simulink model "clrrtsf"  (R2020a)
settings: Solver=FixedStepAuto  StartTime=0.0  StopTime=inf  FixedStep=0.2  RelTol=1e-3
model workspace (MAT data in the model file):
  IC_theta0 : Simulink.Signal (value not decoded)
  IC_x0 : Simulink.Signal (value not decoded)
  IC_x1 : Simulink.Signal (value not decoded)
  IC_y0 : Simulink.Signal (value not decoded)
  IC_y1 : Simulink.Signal (value not decoded)
  contsim_time : Simulink.Signal (value not decoded)
  indicator : Simulink.Signal (value not decoded)
  ip : Simulink.Signal (value not decoded)
  szxx1 : Simulink.Signal (value not decoded)
values from neighbouring files (symbols this model uses):
  indsimtime = 150    [clrrtsf_Initializ.m]
  L_0b = 0.48    [clrrtsf_Initializ.m]    (also in clrrtsolutionplot.m)
  L_0f = 3.8    [clrrtsf_Initializ.m]    (also in clrrtsolutionplot.m)
  L_1f = 7.21    [clrrtsf_Initializ.m]    (also in clrrtsolutionplot.m)
  LD = 10    [clrrtsf_Initializ.m]
  pinit = [80 160 pi 0]    [clrrtsf_Initializ.m]
  tn = zeros(N,14)    [clrrtsf_Initializ.m]    (also in clrrtsolutionplot.m = out.tree)
  veh_path = zeros(indsimtime,6)    [clrrtsf_Initializ.m]
  veh_path_col = zeros(indsimtime,6,N)    [clrrtsf_Initializ.m]
  xx = [-50:0.5:50]'    [clrrtsf_Initializ.m]
  yy = [-50:0.5:50]'    [clrrtsf_Initializ.m]
  Zf = griddata(x,y,znew,xnewt,ynewt)    [clrrtsf_Initializ.m]
  Zr = griddata(x,y,znewr,xnewt,ynewt)    [clrrtsf_Initializ.m]
symbols that are objects in the model workspace (value not decoded): IC_theta0, IC_x0, IC_x1, IC_y0, IC_y1
undefined symbols (not defined in the file or in its folder): DiscIntNeverNeededParam, IC_theta1
libraries: simulink x1
(part 2 of 2)

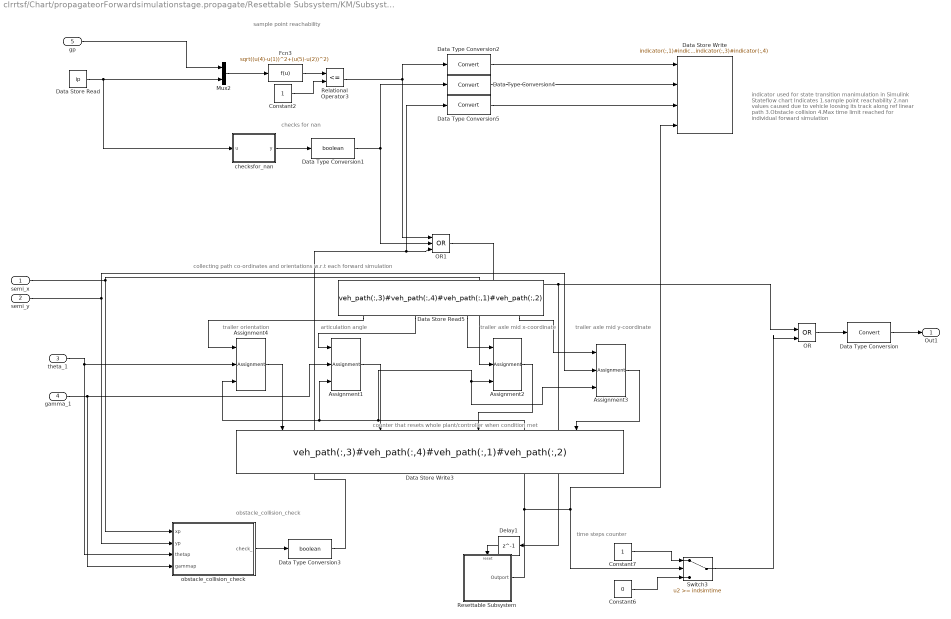
== system clrrtsf/Chart/propagateorForwardsimulationstage.propagate/Resettable Subsystem/KM/Subsystem ==
  note: indicator used for state transition
      | manimulation in Simulink Stateflow chart
      | Indicates
      | 1.sample point reachability
      | 2.nan values caused due to vehicle loosing its track
      | along ref linear path
      | 3.Obstacle collision
      | 4.Max time limit reached for individual forward simulation
  note: collecting path co-ordinates and orientations w.r.t each forward simulation
  note: time steps counter
  note: obstacle_collision_check
  note: counter that resets whole plant/controller when condition met
  note: checks for nan
  note: sample point reachability
  note: trailer axle mid x-coordinate
  note: trailer orientation
  note: articulation angle
  note: trailer axle mid y-coordinate
  semi_x : Inport
  semi_y : Inport  Port=2
  theta_1 : Inport  Port=3
  gamma_1 : Inport  Port=4  OutDataTypeStr=double  PortDimensions=1
  gp : Inport  Port=5
  Assignment{1..4} (4 alike) : Assignment  NumberOfDimensions=2  DiagnosticForDimensions=Warning  IndexOptions=Index vector (port),Index vector (dialog)  Indices=1,1  OutputSizes=1,1
  Constant2 : Constant
  Constant6 : Constant  Value=0
  Constant7 : Constant
  Data Store Read : DataStoreRead  DataStoreName=ip
  Data Store Read5 : DataStoreRead  DataStoreName=veh_path  DataStoreElements=veh_path(:,3)#veh_path(:,4)#veh_path(:,1)#veh_path(:,2)
  Data Store Write : DataStoreWrite  DataStoreName=indicator  DataStoreElements=indicator(:,1)#indicator(:,2)#indicator(:,3)#indicator(:,4)
  Data Store Write3 : DataStoreWrite  DataStoreName=veh_path  DataStoreElements=veh_path(:,3)#veh_path(:,4)#veh_path(:,1)#veh_path(:,2)
  Data Type Conversion{,2,4..5} (4 alike) : DataTypeConversion
  Data Type Conversion1 : DataTypeConversion  OutDataTypeStr=boolean
  Data Type Conversion3 : DataTypeConversion  OutDataTypeStr=boolean
  Delay1 : Delay  DelayLength=1
  Fcn3 : Fcn  Expr=sqrt((u(4)-u(1))^2+(u(5)-u(2))^2)
  Mux2 : Mux  Inputs=2
  OR : Logic  Operator=OR  IconShape=distinctive  AllPortsSameDT=off  OutDataTypeStr=boolean
  OR1 : Logic  Operator=OR  Inputs=3  IconShape=distinctive  AllPortsSameDT=off  OutDataTypeStr=boolean
  Relational Operator3 : RelationalOperator  Operator=<=  OutDataTypeStr=boolean  RndMeth=Simplest
  Resettable Subsystem : Subsystem  TreatAsAtomicUnit=on
  Switch3 : Switch  Threshold=indsimtime
  checksfor_nan : MATLAB Function  TreatAsAtomicUnit=on
  obstacle_collision_check : MATLAB Function  TreatAsAtomicUnit=on
  Out1 : Outport
  wires:
  Delay1/1 -> Resettable Subsystem/Reset
  Assignment2/1 -> Data Store Write3/3
  Constant6/1 -> Switch3/3
  Constant7/1 -> Switch3/1
  OR/1 -> Data Type Conversion/1
  Switch3/1 -> OR/2
  OR1/1 -> OR/1, Delay1/1
  Data Type Conversion/1 -> Out1/1
  semi_x/1 -> obstacle_collision_check/1(xp), Assignment2/2
  Data Store Read5/1 -> Assignment4/1
  Assignment4/1 -> Data Store Write3/1
  theta_1/1 -> obstacle_collision_check/3(thetap), Assignment4/2
  Assignment3/1 -> Data Store Write3/4
  Data Store Read/1 -> checksfor_nan/1(u), Mux2/2
  Fcn3/1 -> Relational Operator3/1
  gp/1 -> Mux2/1
  Constant2/1 -> Relational Operator3/2
  Mux2/1 -> Fcn3/1
  Relational Operator3/1 -> OR1/1, Data Type Conversion2/1
  checksfor_nan/1(y) -> Data Type Conversion1/1
  Data Type Conversion1/1 -> OR1/2, Data Type Conversion4/1
  obstacle_collision_check/1(check_) -> Data Type Conversion3/1
  Data Type Conversion3/1 -> Data Type Conversion5/1, OR1/3
  semi_y/1 -> obstacle_collision_check/2(yp), Assignment3/2
  gamma_1/1 -> obstacle_collision_check/4(gammap), Assignment1/2
  Resettable Subsystem/1(Outport) -> Data Store Write/4, Switch3/2, Assignment1/3, Assignment4/3, Assignment3/3, Assignment2/3
  Data Type Conversion2/1 -> Data Store Write/1
  Data Type Conversion4/1 -> Data Store Write/2
  Data Type Conversion5/1 -> Data Store Write/3
  Assignment1/1 -> Data Store Write3/2
  Data Store Read5/2 -> Assignment1/1
  Data Store Read5/3 -> Assignment2/1
  Data Store Read5/4 -> Assignment3/1

== system clrrtsf/Chart/propagateorForwardsimulationstage.propagate/Resettable Subsystem/KM/Subsystem/Resettable Subsystem ==
  Reset : ResetPort  DisableCoverage=on
  Add1 : Sum
  Constant2 : Constant
  Counter Limited : simulink/Sources/Counter Limited  uplimit=indsimtime-1  tsamp=-1
  Outport : Outport
  wires:
  Counter Limited/1 -> Add1/1
  Constant2/1 -> Add1/2
  Add1/1 -> Outport/1

== matlab function clrrtsf/Chart/stage1.f/For Iterator Subsystem/Subsystem/MATLAB Function1 ==
  data: Nn3 input; localco_ord output size=[1 2]; s input double size=[1 2]; tn data_store_memory
    function localco_ord=coordtransform(Nn3,s)
    global tn
    tnc=tn;
        %theta=90;
        alfa=zeros(1,1);
        if Nn3==1
         %calculating sampled point wrt local coordinates of Nn
            tx = s(1,1);
            ty = s(1,2);
            localco_ord=[tx ty];
        else

            %origin shift and axis rotate
            % - calculate theta is the angle between global X axis and line made by points t(i-1) and t(i)=s()
            % alfa angle btwn global Y axis and line made by points t(i-1) and t(i)=s()
            %            u=(Nn2-tn((Nn3-1),2));
            u=tnc((Nn3),2)- tnc((tnc((Nn3),4)),2);
            v=tnc((Nn3),1)- tnc((tnc((Nn3),4)),1);
            %             v=(Nn1-tn((Nn3-1),1));
            su=sign(u);
            sv=sign(v);
            m=(u)/(v);
            if su >0 && sv>0
                theta=atan(m)*(180/pi);
                alfa = -1*(90 - theta);%cw %270+theta ccw
            elseif su >0 && sv<0
                theta=(atan(m)*(180/pi))+180;    
                alfa=(theta-90);    %ccw
            elseif su <0 && sv<0
                theta=(atan(m)*(180/pi))+180;
                alfa = theta-90; %ccw
            elseif su <0 && sv>0
                theta=(atan(m)*(180/pi))+360; 
                alfa=theta-90; %ccw  %-90-1*(360-theta)cw %
            end
            %calculating sampled point wrt local coordinates of Nn
            tx = (cosd(alfa)*(s(1,1)-tnc((Nn3),1))+sind(alfa)*(s(1,2)-tnc((Nn3),2)));
            ty = (cosd(alfa)*(s(1,2)-tnc((Nn3),2))-sind(alfa)*(s(1,1)-tnc((Nn3),1)));
            localco_ord=[tx ty];
        end
    end

== matlab function clrrtsf/Chart/propagateorForwardsimulationstage.propagate/Resettable Subsystem/Controller/purepursuit_contrroller/func to calculate points of intersections ==
  data: gp input; Nn_ input; tn input; R input; P output; pos input
function P = calc_ips(gp, Nn_, tn, R,pos)
%this func calculates points of intersection between ref line (formed
%with goal point, start point) and look ahead circle with center at semitrailer axel midpoint  
P=zeros(2,2);
%
p1=gp;
p2=[tn(Nn_,1) tn(Nn_,2)];
slope = (p1(1,2)-p2(1,2))/(p1(1,1)-p2(1,1));
if slope == -inf || slope ==inf
    intercpt=p1(1,1);
else
intercpt = p2(1,2)-slope*p2(1,1);
end
%updating center of circle with the current pose of semitrailer axle
%position
centerx=pos(1,1);
centery=pos(2,1);
radius=R;
coder.extrinsic('linecirc')
[xout,yout] = linecirc(slope,intercpt,centerx,centery,radius);
P=[xout ; yout];

== stateflow chart clrrtsf/Chart ==
  note: Implementation of the CL-RRT algorithm in STATEFLOW
  note: START
  state logic for inverting stype variable [group]
    (junction 268) -> (junction 269) [order 1] : [stype==0]
    (junction 268) -> (junction 270) [order 2]
    (junction 269) -> (junction 274) : {stype=1;}
    (junction 270) -> (junction 271) [order 1] : [stype==1]
    (junction 270) -> (junction 272) [order 2]
    (junction 271) -> (junction 273) : {stype=0;}
    (junction 273) -> (junction 272)
    (junction 274) -> (junction 273)
    (junction 272) -> (junction 300) [order 2]
  state stage1
    en:
    %Random sampling when stype is 0
    [sr, v_0]= sampling(i,stype);
    %choosing between nearest and cheapest node with
    % probability of 0.5 for each case
    j=j+1;
    rnum=randnum(j,1);
    if  rnum<=0.5
    %cheapest node finder: f_()
    Nn_= f_(sr,i);
    else
    %Nearest node finder: f()
    Nn_=f(sr,i);
    end
    %Nn_ is the node number of current start point,
    %is uded to index into tree to find respective co-ordinates
    %assigning random sample as current goal point
    gp_(1,1:2)=sr;
    gp_(1,3)=0;%theta;
    % pice wise linear refpath creation between start and
    %goal points
    state Nn = f_(sr,i) [function]
    state Nn = f(sr,i) [function]
  state treebuilder
    i=i+1;   %node increment, where i is the current node number
    j = 0;
    if i==1
    Initialize();
    %initializing vehicle, controller parameters
    %tree, sampling type variable (stype),
    %individual traversedpath, collection of traversed paths
    %insert rootnode into tree
    else
    %parent node number
    pnode=Nn_;
    %m is a function that enters data into the tree array tn
    m(i,pnode,stype,v_0,goalregion);
    %calculating cumulative cost of the traversed path
    cumilativecost(i);
    end
    state cumilativecost(i) [function]
    state Initialize [function]
    state m(i,pnode,stype,f_or_r,goalregion) [function]
  state stage2
    en:
    %goal sampling when stype is 1
    [sg, v_0]= sampling(i,stype);
    % pice wise linear refpath creation
    %assigning goal sample as a
    %next goal point
    gp_(1,1:2)=sg;
    gp_(1,3)=0;%theta;
    %Nn_ is the node number of current
    %start point, is used to index into
    %tree to find respective co-ordinates
    Nn_=i;
    % pice wise linear refpath creation
    % between start and goal points
  state output_to_workspace
    %outputting the tree tn
    %of size Nx14
    %and traversed paths
    %collection in data store
    %with name
    %"Veh_path_col"
    output1wpace();
    state output1wpace [function]
  state updateInitialConfigurationofcontrollerwithNn_
    en:
    %updating the current
    %vehicle position to
    %controller
    updateICofcont(Nn_)
    state updateICofcont(Nn_) [function]
  state goalregion_reachability
    goalregion = goalregionreachability(pgoal);
    %pgoal is the final desired goal pose
    state goalregion = goalregionreachability(pgoal) [function]
  state stopsimulation
  state costcalculation
    en:
    %calculating cost of
    %individual traversed
    % paths by semitrailer
    % driveaxle mid point
    costcal(i);
    state costcal(i) [function]
  state propagateorForwardsimulationstage
    en:
    du:
    propagate(v_0,gp_,Nn_)
    state propagate(v_0,gp,Nn_) [function]
  note: STOP
  note: v_0 & v_1are the logotudinal velocity of tractor and semitrailer set to 1m/s; stype is a variable used to select random sample, (sr) or goal sample, (sg) within the sampling();
      | trans1 is the variable that indicates end of individual forward simulation; Indicator size 1x4 contains boolean values representing true false for sample point reachability, nan
      | values that might result due kinematic infeasibility,obstacle collision and maxtimelimit reach set for each individual forward simulation. Any of these four factors can stop the
      | individual simulation and continue to next; numofnodes is maxlimit on number of nodes
  (default) -> treebuilder : {i=0; rootnode=[190 187 pi 0 0 0 0 0];}
  treebuilder -> (junction 268) [order 2] : [i<numofnodes]
  (junction 272) -> (junction 218) [order 1]
  (junction 218) -> stage1 [order 1] : [ stype == 0]
  (junction 218) -> stage2 [order 2] : [stype == 1]
  treebuilder -> output_to_workspace [order 1] : [i>=numofnodes]
  (junction 242) -> stage1 [order 2] : [(indicator(1,4)<2 && indicator(1,3)==1) || (indicator(1,4)<2 && indicator(1,2)==1) ]
  stage1 -> updateInitialConfigurationofcontrollerwithNn_
  stage2 -> updateInitialConfigurationofcontrollerwithNn_
  output_to_workspace -> stopsimulation
  costcalculation -> treebuilder
  (junction 223) -> treebuilder [order 2] : [i>=numofnodes]
  updateInitialConfigurationofcontrollerwithNn_ -> propagateorForwardsimulationstage
  (junction 223) -> costcalculation [order 1] : [i<numofnodes]
  goalregion_reachability -> (junction 223)
  (junction 242) -> (junction 223) [order 3] : {goalregion=false;}
  (junction 242) -> goalregion_reachability [order 1] : [stype==1 && indicator(1,1)==1]
  propagateorForwardsimulationstage -> (junction 242) : [trans1==1]
  data: sr function_input double size=[1 2]; Nn function_output double; i function_input double size=1; sr function_input double size=[1 2]; Nn function_output double; i function_input double size=1; i function_input double size=[1 1]; i function_input double size=1; pnode function_input double size=1; stype function_input double size=[1 1]; f_or_r function_input double size=[1 1]; goalregion function_input double size=1; in function_input; stype_ function_input; s function_output; v_0_ function_output; Nn_ function_input double size=1; pgoal function_input double size=[1 3]; goalregion function_output; sf_internal_action_state_placeholder_data local double size=1 =0; i function_input double size=[1 1]; v_0 function_input double size=1; gp function_input double size=[1 3]; Nn_ function_input double size=1; tn data_store_memory; sr local size=[1 2]; gp_ local double size=[1 3]; Nn_ local double size=[1 1] =0; i local double size=[1 1] =1; rootnode local; stype local =1; pnode local =0; v_0 data_store_memory; numofnodes data_store_memory =300; sg local; trans1 data_store_memory; pgoal data_store_memory =[0 40 pi/2]; theta local double size=1; indicator data_store_memory; goalregion local; randnum data_store_memory; rnum local; j local
  function [s,v_0_] = sampling(in,stype_):
    | function [s,v_0_] = sampling(in,stype_)
    | %single function called sampling()is used to achive both random sampling ,
    | %(exploring strategy) and goal sampling (biasing strategy). The variable
    | %stype is used to choose the type of the sampling. 0 for random sampling,1
    | %for goal sampling
    | global tn
    | global pgoal
    | global randnum
    | 
    | persistent j
    | if isempty(j)
    | %  costarray=zeros(n,2);
    |  j=0;
    | end
    | j=j+1;
    | tnc=tn;
    | stype=stype_;
    | %rng('shuffle');
    | %rng ( 'default' );
    | while true
    | s=zeros(1,2);
    | v_0_=zeros(1,1);
    | n1=zeros(1,1);
    | refp1=[pgoal(1,1) 145];
    | refp2=[pgoal(1,1) 145];
    |  if stype==0  %random sampling     
    |             %n=rand;
    |             n=randnum(j,1);
    |             if (n>=0)&&(n<=0.2)
    |                 n1=1;
    |             elseif (n>0.2)&&(n<=0.7)
    |                 n1=2;
    |             elseif (n>0.7)&&(n<=1)
    |                 n1=3;
    |             end
    |             switch n1
    |                 case 1
    |                     %forward
    |                     sigmaU=[5,5];
    |                     %s(1,1)=tn(in,1)+ sqrt(3)*sigmaU(1)*(-1+2.*rand); %-1+2.*
    |                     s(1,1)=refp2(1,1)+ sqrt(3)*sigmaU(1)*(-1+2.*rand);
    |                     %s(1,2)=tn(in,2)+ sqrt(3)*sigmaU(2)*(-1+2.*rand); %-1+2.*
    |                     s(1,2)=refp2(1,2)+ sqrt(3)*sigmaU(2)*(-1+2.*rand);
    |                     v_0_=-1;
    |                 case 2
    |                     sigmaU=[2.5,5];
    |                     %s(1,1)=tn(in,1)+ sqrt(3)*sigmaU(1)*(-1+2.*rand); %-1+2.*
    |                     s(1,1)=refp2(1,1)+ sqrt(3)*sigmaU(1)*(-1+2.*rand);
    |                     %s(1,2)=tn(in,2)+ sqrt(3)*sigmaU(2)*(-1+2.*rand); %-1+2.*
    |                     s(1,2)=refp2(1,2)+ sqrt(3)*sigmaU(2)*(-1+2.*rand);
    |                     v_0_=-1;
    |                 case 3
    |                     sigmaU=[2.5,5];
    |                     %s(1,1)=tn(in,1)+ sqrt(3)*sigmaU(1)*(-1+2.*rand); %-1+2.*
    |                     s(1,1)=refp1(1,1)+ sqrt(3)*sigmaU(1)*(-1+2.*rand);
    |                     %s(1,2)=tn(in,2)+ sqrt(3)*sigmaU(2)*(-1+2.*rand); %-1+2.*
    |                     s(1,2)=refp1(1,2)+ sqrt(3)*sigmaU(2)*(-1+2.*rand);
    |                     v_0_=-1;
    | 
    |             end
    | 
    |  elseif stype==1       %goal sampling   
    | 
    |             
    |                        % pgoal=[0 40 pi/2];
    |             R=10;
    |             sigmaR=R/35;
    |             goaltheta=pgoal(1,3);
    |             sigmaTheta=pi/40000;
    |             r=sqrt(3)*sigmaR*(-1*randnum(j,1))+(-1*R);%(sign(v_0_)*R); 
    |             theta=sqrt(3)*sigmaTheta*(-1+2.*randnum(j,1))+goaltheta;
    |             s(1,1)=pgoal(1,1)+r*cos(theta);
    |             s(1,2)=pgoal(1,2)+r*sin(theta);
    |             v_0_=-1;
    |         
    |  end
    |   
    |  % %region1
    | % refpoint - [120 150]
    | % sigmaU=[20,15];
    | % sigmaU=[35,15];
    | %  sigmaU=[20,15];
    |  
    |  % %region2
    | % pgoal=[170 193 pi]; pinit=[190 187 pi];
    | % refpoint - [170 185]
    | % sigmaU=[20,10];
    | % sigmaU=[35,5];
    | %  sigmaU=[35,10];
    | 
    | % %region3
    | %all rev direction
    | % pgoal=[202.4 71.5 (3*pi)/4]; pinit=[230 50 0];
    | % refp=[215 50];
    | %refp2=[pgoal(1,1)+6 50];
    | % sigmaU=[10,10];
    | % sigmaU=[5,5];
    | %  sigmaU=[5,15];
    | % R=10;
    | %             sigmaR=R/35;
    | %             goaltheta=pgoal(1,3);
    | %             sigmaTheta=pi/40000;
    | %             r=sqrt(3)*sigmaR*(-1*randnum(j,1))+(-1*R);%(sign(v_0_)*R); 
    | %             theta=sqrt(3)*sigmaTheta*(-1+2.*randnum(j,1))+goaltheta;
    | 
    | % 
    | % case 1
    | %                     %forward
    | %                     sigmaU=[24.7,24.7];
    | %                     %s(1,1)=tn(in,1)+ sqrt(3)*sigmaU(1)*(-1+2.*rand); %-1+2.*
    | %                     s(1,1)=175+ sqrt(3)*sigmaU(1)*(-1+2.*rand);
    | %                     %s(1,2)=tn(in,2)+ sqrt(3)*sigmaU(2)*(-1+2.*rand); %-1+2.*
    | %                     s(1,2)=187+ sqrt(3)*sigmaU(2)*(-1+2.*rand);
    | %                     v_0_=1;
    | %                 case 2
    | %                     sigmaU=[16.4,16.4];
    | %                     %s(1,1)=tn(in,1)+ sqrt(3)*sigmaU(1)*(-1+2.*rand); %-1+2.*
    | %                     s(1,1)=175+ sqrt(3)*sigmaU(1)*(-1+2.*rand);
    | %                     %s(1,2)=tn(in,2)+ sqrt(3)*sigmaU(2)*(-1+2.*rand); %-1+2.*
    | %                     s(1,2)=187+ sqrt(3)*sigmaU(2)*(-1+2.*rand);
    | %                     v_0_=1;
    | %                 case 3
    | %                     sigmaU=[25,25];
    | %                     %s(1,1)=tn(in,1)+ sqrt(3)*sigmaU(1)*(-1+2.*rand); %-1+2.*
    | %                     s(1,1)=175+ sqrt(3)*sigmaU(1)*(-1+2.*rand);
    | %                     %s(1,2)=tn(in,2)+ sqrt(3)*sigmaU(2)*(-1+2.*rand); %-1+2.*
    | %                     s(1,2)=187+ sqrt(3)*sigmaU(2)*(-1+2.*rand);
    | %                     v_0_=1;
    | 
    | 
    | %%
    | %  case 1
    | %                     %forward
    | %                     sigmaU=[75,70];%[24.7,10];
    | %                     %s(1,1)=tn(in,1)+ sqrt(3)*sigmaU(1)*(-1+2.*rand); %-1+2.*
    | %                     s(1,1)=150+ sqrt(3)*sigmaU(1)*(-1+2.*rand);
    | %                     %s(1,2)=tn(in,2)+ sqrt(3)*sigmaU(2)*(-1+2.*rand); %-1+2.*
    | %                     s(1,2)=100+ sqrt(3)*sigmaU(2)*(-1+2.*rand);
    | %                     v_0_=1;
    | %                 case 2
    | %                     sigmaU=[38,25];%[16 16]
    | %                     %s(1,1)=tn(in,1)+ sqrt(3)*sigmaU(1)*(-1+2.*rand); %-1+2.*
    | %                     s(1,1)=175+ sqrt(3)*sigmaU(1)*(-1+2.*rand);
    | %                     %s(1,2)=tn(in,2)+ sqrt(3)*sigmaU(2)*(-1+2.*rand); %-1+2.*
    | %                     s(1,2)=187+ sqrt(3)*sigmaU(2)*(-1+2.*rand);
    | %                     v_0_=1;
    | %                 case 3
    | %                     sigmaU=[75,70];
    | %                     %s(1,1)=tn(in,1)+ sqrt(3)*sigmaU(1)*(-1+2.*rand); %-1+2.*
    | %                     s(1,1)=150+ sqrt(3)*sigmaU(1)*(-1+2.*rand);
    | %                     %s(1,2)=tn(in,2)+ sqrt(3)*sigmaU(2)*(-1+2.*rand); %-1+2.*
    | %                     s(1,2)=100+ sqrt(3)*sigmaU(2)*(-1+2.*rand);
    | %                     v_0_=1;
    | 
    | 
    | 
    |  break
    |         
    | end
    | 
    | %             %v_0_ for gsample
    | %             alfa=zeros(1,1);
    | %             if in==1
    | %              %calculating goal point wrt local coordinates of Nn
    | %                 tx = pgoal(1,1);
    | %                 ty = pgoal(1,2);
    | %                 if ty>0
    | %                     v_0_=1;
    | %                 else
    | %                     v_0_=-1;
    | %                 end
    | %             else
    | %                 theta_=tn(in,9)*(180/pi);
    | %                 if theta_ >=0 && theta_<=90       %1st quad                  
    | %                     alfa = -1*(90 - theta_);%cw %270+theta_ ccw
    | %                 elseif theta_ > 90 && theta_<=180   %2nd quad   
    | %                     alfa=(theta_-90);    %ccw
    | %                 elseif theta_>180 && theta_<=270   %3rd quad
    | %                     alfa = theta_-90; %ccw
    | %                 elseif theta_>270 && theta_<=360   %4th quad
    | %                     alfa=theta_-90; %ccw  %-90-1*(360-theta_)cw %
    | %                 end
    | %                 %calculating pgoal point wrt local coordinates of Nn
    | %                 tx = (cosd(alfa)*(pgoal(1,1)-tnc((in),1))+sind(alfa)*(pgoal(1,2)-tnc((in),2)));
    | %                 ty = (cosd(alfa)*(pgoal(1,2)-tnc((in),2))-sind(alfa)*(pgoal(1,1)-tnc((in),1)));
    | %                 if ty>0
    | %                     v_0_=1;
    | %                 else
    | %                     v_0_=-1;
    | %                 end
    | %             end
    | 
    | 
    | %region4
    | % refp1=[pgoal(1,1) 145];
    | % refp2=[pgoal(1,1)-6 160];
    | %  if stype==0  %random sampling     
    | %             %n=rand;
    | %             n=randnum(j,1);
    | %             if (n>=0)&&(n<=0.2)
    | %                 n1=1;
    | %             elseif (n>0.2)&&(n<=0.7)
    | %                 n1=2;
    | %             elseif (n>0.7)&&(n<=1)
    | %                 n1=3;
    | %             end
    | %             switch n1
    | %                 case 1
    | %                     %forward
    | %                     sigmaU=[5,5];
    | %                     %s(1,1)=tn(in,1)+ sqrt(3)*sigmaU(1)*(-1+2.*rand); %-1+2.*
    | %                     s(1,1)=refp2(1,1)+ sqrt(3)*sigmaU(1)*(-1+2.*rand);
    | %                     %s(1,2)=tn(in,2)+ sqrt(3)*sigmaU(2)*(-1+2.*rand); %-1+2.*
    | %                     s(1,2)=refp2(1,2)+ sqrt(3)*sigmaU(2)*(-1+2.*rand);
    | %                     v_0_=-1;
    | %                 case 2
    | %                     sigmaU=[2.5,5];
    | %                     %s(1,1)=tn(in,1)+ sqrt(3)*sigmaU(1)*(-1+2.*rand); %-1+2.*
    | %                     s(1,1)=refp2(1,1)+ sqrt(3)*sigmaU(1)*(-1+2.*rand);
    | %                     %s(1,2)=tn(in,2)+ sqrt(3)*sigmaU(2)*(-1+2.*rand); %-1+2.*
    | %                     s(1,2)=refp2(1,2)+ sqrt(3)*sigmaU(2)*(-1+2.*rand);
    | %                     v_0_=-1;
    | %                 case 3
    | %                     sigmaU=[2.5,12];
    | %                     %s(1,1)=tn(in,1)+ sqrt(3)*sigmaU(1)*(-1+2.*rand); %-1+2.*
    | %                     s(1,1)=refp1(1,1)+ sqrt(3)*sigmaU(1)*(-1+2.*rand);
    | %                     %s(1,2)=tn(in,2)+ sqrt(3)*sigmaU(2)*(-1+2.*rand); %-1+2.*
    | %                     s(1,2)=refp1(1,2)+ sqrt(3)*sigmaU(2)*(-1+2.*rand);
    | %                     v_0_=-1;
    | % 
    | %             end
    | % 
    | %  elseif stype==1       %goal sampling   
    | % 
    | %             
    | %                        % pgoal=[0 40 pi/2];
    | %             R=10;
    | %             sigmaR=R/35;
    | %             goaltheta=pgoal(1,3);
    | %             sigmaTheta=pi/40000;
    | %             r=sqrt(3)*sigmaR*(-1*randnum(j,1))+(-1*R);%(sign(v_0_)*R); 
    | %             theta=sqrt(3)*sigmaTheta*(-1+2.*randnum(j,1))+goaltheta;
    | %             s(1,1)=pgoal(1,1)+r*cos(theta);
    | %             s(1,2)=pgoal(1,2)+r*sin(theta);
    | %             v_0_=-1;
    | %

== matlab function clrrtsf/Chart/stage1.f/For Iterator Subsystem/MATLAB Function ==
  data: i input; cost input size=[1 1]; sztn data_store_memory; i_ input; Nn output size=[1 1]
function Nn = fcn(i, cost, i_)

%finding nearest neighbour based on Heuristic map cost data
persistent costarray
Nn=1;
% coder
if isempty(costarray)
%  costarray=zeros(n,2);
 costarray=zeros(i_,2);
end

costarray(i,1)=i; %node num
costarray(i,2)=cost;
if i == i_
 so_costarray=sortrows(costarray,2);
%  szso_co=size(so_costarray,1);
 for j=1:i_%szso_co
     if so_costarray(j,2)~=0
     Nn=so_costarray(j,1);
     break
     end
 end
        
end

== matlab function clrrtsf/Chart/propagateorForwardsimulationstage.propagate/Resettable Subsystem/Controller/purepursuit_contrroller/pure pursuit control law ==
  data: ip output; P input size=[2 2]; alpha output size=[1,1]; gp input size=[1 3]; L_1f input; yawangle_semi input; pos input; R input
function [ip,alpha] = controlleroutput(P,gp,L_1f,yawangle_semi,pos,R)
%this func calculates steer angle that pursues the ref line formed between
%start point and goal point chosen from wayp

Psz=size(P,2);          %num of intersection points, with x_cords in 1st column y_cords in 2nd column in matrix P
distarray=zeros(Psz,3); % intersection points distance to gp (goal point)
 for k=1:Psz
     distarray(k,1:2)=[P(1,k) P(2,k)];
     distarray(k,3)=sqrt((P(1,k)-gp(1,1))^2+(P(2,k)-gp(1,2))^2);
 end
%choosing the nearest intersection point to the goal point from the
%available 2 points of intersection between reference line and look ahead
%circle
sortP=sortrows(distarray,3);  
ip=sortP(1,1:2);
alpha=zeros(1,1);
%Theta_e
num=ip(1,1)-pos(1,1);
den=ip(1,2)-pos(2,1);
theta_e = atan2(den,num)-yawangle_semi;   %orientation error
alpha = -atan((2*L_1f*sin(theta_e))/R);   %steer angle that aims to reduce orientation error (please refer the thesis doc for graphical explaination)

== matlab function clrrtsf/Chart/updateInitialConfigurationofcontrollerwithNn_.updateICofcont/MATLAB Function ==
  data: IC_x1 output; IC_y1 output; Nn_ input; IC_x0 output; tn input; IC_y0 output; IC_theta0 output; IC_theta1 output
function [IC_x1,IC_y1,IC_x0,IC_y0,IC_theta0,IC_theta1] = fcn(Nn_,tn)
%semitraileraxle x and y states; semitrailer orientation theta_1;
%articulation angle gamma_1; gamma_1=theta_0-theta_1;
Nn=[tn(Nn_,1) tn(Nn_,2) tn(Nn_,9) tn(Nn_,10)];
L_0f = 3.8;  %(tractor wheelbase)
L_1f = 7.21; %(trailer wheel base)
L_0b = 0.48;
        %updating the vehicle position to controller
                IC_x1= 0+Nn(1,1);                                                         % initial x-position of semi axle 
                IC_y1 = 0+Nn(1,2);
                IC_theta1 = Nn(1,3);
                IC_theta0 = Nn(1,4)+Nn(1,3);                                                   % initial yaw angle of tractor [deg]
                
                
                IC_x1f= L_1f*cos(IC_theta1)+IC_x1 ;                                                         % initial x-position of semi axle 
                IC_y1f =L_1f*sin(IC_theta1)+IC_y1 ;
                
                IC_x0f= (L_0f-L_0b)*cos(IC_theta0)+IC_x1f ;                                                         % initial x-position of semi axle 
                IC_y0f =(L_0f-L_0b)*sin(IC_theta0)+IC_y1f ;
                
                IC_x0 =   IC_x0f-L_0f*cos(IC_theta0);                                                           % initial x-position of tractor drive axle 
                IC_y0 =   IC_y0f-L_0f*sin(IC_theta0);

== matlab function clrrtsf/Chart/costcalculation.costcal/MATLAB Function ==
  data: veh_path input; costt output
function costt =costfun(veh_path)
%         costt = 0;
%         temp = 0;
        costt=0;
        totalsteps=length(veh_path(:,:));
        for m = 2:totalsteps
        temp = (10*(veh_path(m,1)-veh_path(m-1,1))^2+10*(veh_path(m,2)-veh_path(m-1,2))^2);   %based on "Motion Planning and Stabilization for a Reversing Truck and Trailer System" Oskar Ljungqvist
        costt = costt + temp;
        end

end

== matlab function clrrtsf/Chart/treebuilder.cumilativecost/MATLAB Function ==
  data: tn input; totallen output; i input
function totallen =cumilativecost(tn,i)
if i~=1
%calculates the cumulative cost, by adding each individual extension cost
% calculated by function costcal() a state in the simulink statflow. 
%This is done by tracing back from current node tn(i,3) 
%to the root node that is the initial point pinit, Currnt node is considered
%child node and its parentnode as the previous node that the current node can
% trace back 
        childnoden=tn(i,3);
        childnodepn=tn(i,4);
        totallen=0;
        xx=0;
        while true
            %traj length between childnode and patrent node
            xx=xx+tn(childnoden,6);
            b=childnodepn;
            parentnoden=tn(b,3);
            parentnodepn=tn(b,4);
            %current parentnode will be next steps childnode
            childnoden=parentnoden;
            childnodepn=parentnodepn;
            if b==1
                totallen=xx;
                break
            end
        end
else
    totallen=0;
end

== matlab function clrrtsf/Chart/propagateorForwardsimulationstage.propagate/Resettable Subsystem/IK/IK_function ==
  data: x_1 input; y_1 input; theta_0 input; theta_1 input; x_1_dot output; gamma_virtual input; y_1_dot output; theta_0_dot output; theta_1_dot output; v_1 input; x_0f output; y_0f output; x_0 output; y_0 output; x_1f output; y_1f output; delta_C input; delta_I2K output; v_0 input
% The vehicle is described in global coordinates for which ISO system is used.
% Yaw rates can be derived from applying non-holonomic consraint (no lateral
% slip) on each axle.

function [x_1_dot,y_1_dot,theta_0_dot,theta_1_dot,x_0f,y_0f,x_0,y_0,x_1f,y_1f,...
         delta_I2K] = vehicle(x_1,y_1,theta_0,theta_1,gamma_virtual,v_1,delta_C, v_0)
     
L_0f = 3.8;  %(tractor wheelbase)
L_1f = 7.21; %(trailer wheel base)
L_0b = 0.48;
     %_______________________ position _________________________________________
%king-pin

        x_1f = x_1+L_1f*cos(theta_1);
        y_1f = y_1+L_1f*sin(theta_1);

 
% drive axle

        x_0 = x_1f-L_0b*cos(theta_0);
        y_0 = y_1f-L_0b*sin(theta_0);

% steer axle

        x_0f = x_0+L_0f*cos(theta_0);
        y_0f = y_0+L_0f*sin(theta_0);
                       
% yaw rate        
                                      
        theta_1_dot = abs(v_1)*tan(delta_C)/L_1f;                           % semitrailer
        theta_0_dot = sign(v_1)*sign(L_0b)*(-(v_1/L_0b)*sin(gamma_virtual)+...
                    (L_1f/L_0b)*(theta_1_dot)*cos(gamma_virtual));                % tractor 
                     
% semitrailer longitudinal velocity in its own local body coordinate system

       
        
        delta_I2K = atan(L_0f*theta_0_dot/v_0);
                    
        
%_________________________next iteration___________________________________
        
        x_1_dot = v_1 * cos(theta_1);                                       % tractor drive axle velocity in global x-direction
        y_1_dot = v_1 * sin(theta_1);                                       % tractor drive axle velocity in global y-direction

== matlab function clrrtsf/Chart/propagateorForwardsimulationstage.propagate/Resettable Subsystem/KM/KM function ==
  data: x_0 input; y_0 input; theta_0 input; theta_1 input; x_0_dot output; L_0b parameter; L_1f parameter; y_0_dot output; theta_0_dot output; theta_1_dot output; v_0 input; x_0f output; y_0f output; x_1f output; y_1f output; x_1 output; y_1 output; gamma_1 output; v_1 output; delta input; L_0f parameter
% The vehicle is described in global coordinates for which ISO system is used.
% Yaw rates can be derived from applying non-holonomic consraint (no lateral
% slip) on each axle.

function [x_0_dot,y_0_dot,theta_0_dot,theta_1_dot,x_0f,y_0f,x_1f,y_1f,x_1,y_1,gamma_1,...
         v_1] = vehicle(x_0,y_0,theta_0,theta_1,L_0b, L_1f, v_0,delta, L_0f)
     
%_______________________ position _________________________________________
% steer axle

        x_0f = x_0+L_0f*cos(theta_0);
        y_0f = y_0+L_0f*sin(theta_0);
        
%king-pin

        x_1f = x_0+L_0b*cos(theta_0);
        y_1f = y_0+L_0b*sin(theta_0);
 
% semitrailer axle

        x_1 = x_1f-L_1f*cos(theta_1);
        y_1 = y_1f-L_1f*sin(theta_1);
        
% articulation angle
        
        gamma_1 = (theta_0-theta_1);                                        % articulation angle
        
% yaw rate        
        
        theta_0_dot = (v_0/L_0f) * tan(delta);                              % tractor 
        theta_1_dot = (v_0/L_1f)*sin(gamma_1) + (L_0b/L_1f)*...
                        (theta_0_dot)*cos(gamma_1);                         % semitrailer                            
                    
                    
% semitrailer longitudinal velocity in its own local body coordinate system

        v_1 = 1;  
                    
        
%_________________________next iteration____________________________________
        
        x_0_dot = v_0 * cos(theta_0);                                          % tractor drive axle velocity in global x-direction
        y_0_dot = v_0 * sin(theta_0);                                          % tractor drive axle velocity in global y-direction

== matlab function clrrtsf/Chart/propagateorForwardsimulationstage.propagate/Subsystem/Subsystem1/MATLAB Function ==
  data: veh_path input; y output size=[1 8]; gp input
function y = fcn(veh_path, gp)
%to obtain the final co-ordinates after respective forward simulation
y=zeros(1,8);
x=find(veh_path(:,1), 1, 'last' );
x1=x(1,1);
y=[veh_path(x1,1:6) gp(1,1:2)];%last two places have sample co-ordinates

== matlab function clrrtsf/Chart/stage1.f_/For Iterator Subsystem/MATLAB Function ==
  data: i input; cost input size=[1 1]; sztn data_store_memory; i_ input; Nn output size=[1 1]; tn data_store_memory
function Nn = fcn(i, cost, i_)
%finding the cheapest node based on the cost data from the heuristic maps
%and cumulative cost combination
global tn
% global sztn
persistent costarray
Nn=1;
% coder
if isempty(costarray)
 costarray=zeros(i_,2);
end
%traversed path length stored in global data store tn(i,7)of the node "i" in consideration
costarray(i,1)=i; %node num
costarray(i,2)=cost+tn(i,7);
if i == i_
 so_costarray=sortrows(costarray,2);
%  szso_co=size(so_costarray,1);
 for j=1:i_%szso_co
     if so_costarray(j,2)~=0
     Nn=so_costarray(j,1);
     break
     end
 end
        
end

== matlab function clrrtsf/Chart/stage1.f_/For Iterator Subsystem/Subsystem/MATLAB Function1 ==
  data: Nn3 input; localco_ord output size=[1 2]; s input double size=[1 2]; tn data_store_memory
    function localco_ord=coordtransform(Nn3,s)
    global tn
    tnc=tn;
        %theta=90;
        alfa=zeros(1,1);
        if Nn3==1
         %calculating sampled point wrt local coordinates of Nn
            tx = s(1,1);
            ty = s(1,2);
            localco_ord=[tx ty];
        else

            %origin shift and axis rotate
            % - calculate theta is the angle between global X axis and line made by points t(i-1) and t(i)=s()
            % alfa angle btwn global Y axis and line made by points t(i-1) and t(i)=s()
            %            u=(Nn2-tn((Nn3-1),2));
            u=tnc((Nn3),2)- tnc((tnc((Nn3),4)),2);
            v=tnc((Nn3),1)- tnc((tnc((Nn3),4)),1);
            %             v=(Nn1-tn((Nn3-1),1));
            su=sign(u);
            sv=sign(v);
            m=(u)/(v);
            if su >0 && sv>0
                theta=atan(m)*(180/pi);
                alfa = -1*(90 - theta);%cw %270+theta ccw
            elseif su >0 && sv<0
                theta=(atan(m)*(180/pi))+180;    
                alfa=(theta-90);    %ccw
            elseif su <0 && sv<0
                theta=(atan(m)*(180/pi))+180;
                alfa = theta-90; %ccw
            elseif su <0 && sv>0
                theta=(atan(m)*(180/pi))+360; 
                alfa=theta-90; %ccw  %-90-1*(360-theta)cw %
            end
            %calculating sampled point wrt local coordinates of Nn
            tx = (cosd(alfa)*(s(1,1)-tnc((Nn3),1))+sind(alfa)*(s(1,2)-tnc((Nn3),2)));
            ty = (cosd(alfa)*(s(1,2)-tnc((Nn3),2))-sind(alfa)*(s(1,1)-tnc((Nn3),1)));
            localco_ord=[tx ty];
        end
    end

== matlab function clrrtsf/Chart/stage1.f_/For Iterator Subsystem/Subsystem1/MATLAB Function1 ==
  data: Nn3 input; localco_ord output size=[1 2]; s input double size=[1 2]; tn data_store_memory
    function localco_ord=coordtransform(Nn3,s)
    global tn
    tnc=tn;
        %theta=90;
        alfa=zeros(1,1);
        if Nn3==1
         %calculating sampled point wrt local coordinates of Nn
            tx = s(1,1);
            ty = s(1,2);
            localco_ord=[tx ty];
        else

            %origin shift and axis rotate
            % - calculate theta is the angle between global X axis and line made by points t(i-1) and t(i)=s()
            % alfa angle btwn global Y axis and line made by points t(i-1) and t(i)=s()
            %            u=(Nn2-tn((Nn3-1),2));
            u=tnc((Nn3),2)- tnc((tnc((Nn3),4)),2);
            v=tnc((Nn3),1)- tnc((tnc((Nn3),4)),1);
            %             v=(Nn1-tn((Nn3-1),1));
            su=sign(u);
            sv=sign(v);
            m=(u)/(v);
            if su >0 && sv>0
                theta=atan(m)*(180/pi);
                alfa = -1*(90 - theta);%cw %270+theta ccw
            elseif su >0 && sv<0
                theta=(atan(m)*(180/pi))+180;    
                alfa=(theta-90);    %ccw
            elseif su <0 && sv<0
                theta=(atan(m)*(180/pi))+180;
                alfa = theta-90; %ccw
            elseif su <0 && sv>0
                theta=(atan(m)*(180/pi))+360; 
                alfa=theta-90; %ccw  %-90-1*(360-theta)cw %
            end
            %calculating sampled point wrt local coordinates of Nn
            tx = (cosd(alfa)*(s(1,1)-tnc((Nn3),1))+sind(alfa)*(s(1,2)-tnc((Nn3),2)));
            ty = (cosd(alfa)*(s(1,2)-tnc((Nn3),2))-sind(alfa)*(s(1,1)-tnc((Nn3),1)));
            localco_ord=[tx ty];
        end
    end

== matlab function clrrtsf/Chart/stage1.f/For Iterator Subsystem/Subsystem1/MATLAB Function1 ==
  data: Nn3 input; localco_ord output size=[1 2]; s input double size=[1 2]; tn data_store_memory
    function localco_ord=coordtransform(Nn3,s)
    global tn
    tnc=tn;
        %theta=90;
        alfa=zeros(1,1);
        if Nn3==1
         %calculating sampled point wrt local coordinates of Nn
            tx = s(1,1);
            ty = s(1,2);
            localco_ord=[tx ty];
        else

            %origin shift and axis rotate
            % - calculate theta is the angle between global X axis and line made by points t(i-1) and t(i)=s()
            % alfa angle btwn global Y axis and line made by points t(i-1) and t(i)=s()
            %            u=(Nn2-tn((Nn3-1),2));
            u=tnc((Nn3),2)- tnc((tnc((Nn3),4)),2);
            v=tnc((Nn3),1)- tnc((tnc((Nn3),4)),1);
            %             v=(Nn1-tn((Nn3-1),1));
            su=sign(u);
            sv=sign(v);
            m=(u)/(v);
            if su >0 && sv>0
                theta=atan(m)*(180/pi);
                alfa = -1*(90 - theta);%cw %270+theta ccw
            elseif su >0 && sv<0
                theta=(atan(m)*(180/pi))+180;    
                alfa=(theta-90);    %ccw
            elseif su <0 && sv<0
                theta=(atan(m)*(180/pi))+180;
                alfa = theta-90; %ccw
            elseif su <0 && sv>0
                theta=(atan(m)*(180/pi))+360; 
                alfa=theta-90; %ccw  %-90-1*(360-theta)cw %
            end
            %calculating sampled point wrt local coordinates of Nn
            tx = (cosd(alfa)*(s(1,1)-tnc((Nn3),1))+sind(alfa)*(s(1,2)-tnc((Nn3),2)));
            ty = (cosd(alfa)*(s(1,2)-tnc((Nn3),2))-sind(alfa)*(s(1,1)-tnc((Nn3),1)));
            localco_ord=[tx ty];
        end
    end

== matlab function clrrtsf/Chart/propagateorForwardsimulationstage.propagate/Resettable Subsystem/KM/Subsystem/checksfor_nan ==
  data: u input; y output
function y = fcn(u)
if any(isnan(u), 'all')
    y=1;
else
    y=0;
end

== matlab function clrrtsf/Chart/propagateorForwardsimulationstage.propagate/Resettable Subsystem/KM/Subsystem/obstacle_collision_check ==
  data: xp input; check_ output; yp input; thetap input; gammap input; obs data_store_memory
function check_ = obs_check_(xp,yp,thetap,gammap)
% global vehicle_paths
global obs
obsc=size(obs,1);
obsx=obs(:,:,1);
obsy=obs(:,:,2);
check_=0;     % Collision check_ variable %0 is no collision; 1 is collided with obstacle
% xp=vehicle_paths(:,1,i_);
% yp=vehicle_paths(:,2,i_);
% thetap=vehicle_paths(:,3,i_);
% gammap=vehicle_paths(:,4,i_);
% We have the position of the trailer axle(xp,yp) and the orientation of the
% trailer(thetap) and the articulation angle (gammap). So from all this
% information we can find all the four corners of the trailer and the four
% corners of the tractor and see if these corners are hitting the obstacle.
%%
L_0f = 3.8;  %(tractor wheelbase)
L_1f = 7.21; %(trailer wheel base)
L_0b = 0.48;  %% Distance of 1st king-pin to tractor drive axle [m][m]
oh_1b = 4.3260;       % Longitudinal distance from the trailer axle to the end of the trailer [m] (60% of the WB)
oh_1f = L_1f+1;  % Longitudinal distance from the trailer axle to the front of the trailer [m]
w_1   = 2.5;     % Width of a trailer [m]
% Now  we will create vectors to each corner of the trailer
% Length of vector 1, 2 is the same and 3,4 is the same
lv12_1 = hypot(oh_1b,(w_1/2)); % Length of Vector 1 and 2
lv34_1 = hypot((w_1/2),oh_1f); % Length of Vector 3 and 4
% if dirp == 0
%     thetap=thetap+deg2rad(180);
%     thetap=wrapTo360(thetap);
%     gammap= -gammap;
% end

% Now we have to find the corners of the tractor. The tractor and the
% trailer have one point the same and fixed which is the king pin.

oh_0f = 1.5; % Frontal foverhang of the truck [m
oh_0b = 0.94; % Distance from the drive axle to the end of the tractor [m]
lv12_0 = hypot((oh_0b),(w_1/2)); % Length of Vector 1 and 2
lv34_0 = hypot((w_1/2),(L_0f+oh_0f)); % Length of Vector 3 and 4

% For Trailer
% Angle of the vectors
av1 = (180/pi*thetap)+90+atand(oh_1b/(w_1/2)); % Angle of Vector 1
av2 = (180/pi*thetap)-90-atand(oh_1b/(w_1/2)); % Angle of Vector 2
av3 = (180/pi*thetap)-atand((w_1/2)/oh_1f); % Angle of Vector 3
av4 = (180/pi*thetap)+atand((w_1/2)/oh_1f); % Angle of Vector 4

% Finding the corner points of the trailer at every (xp,yp)
xv1_1 = xp+lv12_1*cosd(av1);
yv1_1 = yp+lv12_1*sind(av1);
xv2_1 = xp+lv12_1*cosd(av2);
yv2_1 = yp+lv12_1*sind(av2);
xv3_1 = xp+lv34_1*cosd(av3);
yv3_1 = yp+lv34_1*sind(av3);
xv4_1 = xp+lv34_1*cosd(av4);
yv4_1 = yp+lv34_1*sind(av4);

%For tractor
x_1f = xp+L_1f*cos(thetap); % Position of the king pin
y_1f = yp+L_1f*sin(thetap);
theta_0 = thetap+gammap; % Orientation angle of tractor [rad]
x_0 = x_1f-L_0b*cos(theta_0); % Position of center of the driven axle
y_0 = y_1f-L_0b*sin(theta_0);
% Angle of the vectors
av1 = (180/pi*(theta_0))+90+atand(oh_0b/(w_1/2)); % Angle of Vector 1
av2 = (180/pi*(theta_0))-90-atand(oh_0b/(w_1/2)); % Angle of Vector 2
av3 = (180/pi*(theta_0))-atand((w_1/2)/(oh_0f+L_0f)); % Angle of Vector 3
av4 = (180/pi*(theta_0))+atand((w_1/2)/(oh_0f+L_0f)); % Angle of Vector 4

% Finding the corner points of tractor at every (xp,yp)
xv1_0 = x_0+lv12_0*cosd(av1);
yv1_0 = y_0+lv12_0*sind(av1);
xv2_0 = x_0+lv12_0*cosd(av2);
yv2_0 = y_0+lv12_0*sind(av2);
xv3_0 = x_0+lv34_0*cosd(av3);
yv3_0 = y_0+lv34_0*sind(av3);
xv4_0 = x_0+lv34_0*cosd(av4);
yv4_0 = y_0+lv34_0*sind(av4);

xc=[xv1_1;xv2_1;xv3_1;xv4_1;xv1_0;xv2_0;xv3_0;xv4_0];
yc=[yv1_1;yv2_1;yv3_1;yv4_1;yv1_0;yv2_0;yv3_0;yv4_0];

cibxmax= any(xc>=286);
cibymax= any(yc>=200);
cibxmin= any(xc<=0);
cibymin= any(yc<=0);



    for j=1:obsc
        obsxtemp=obsx(j,:);
        obsytemp=obsy(j,:);
        obsxtemp=obsxtemp(obsxtemp~=0);
        obsytemp=obsytemp(obsytemp~=0);
        in1 = inpolygon(xc,yc,obsxtemp,obsytemp); % check_ whether cur is hitting obs
        in1 = any(in1);
        if in1 == 1 ||cibxmax==1||cibymax==1||cibxmin==1||cibymin==1
         check_ = 1; %1 is collided with obstacle
         break;
        end
    end


end

== matlab function clrrtsf/Chart/propagateorForwardsimulationstage.propagate/Enabled Subsystem/MATLAB Function ==
  data: IC_x1 output; IC_y1 output; Nn_ input; IC_x0 output; tn input; IC_y0 output; IC_theta0 output; IC_theta1 output
function [IC_x1,IC_y1,IC_x0,IC_y0,IC_theta0,IC_theta1] = fcn(Nn_,tn)
%semitraileraxle x and y states; semitrailer orientation theta_1;
%articulation angle gamma_1; gamma_1=theta_0-theta_1;
Nn=[tn(Nn_,1) tn(Nn_,2) tn(Nn_,9) tn(Nn_,10)];
L_0f = 3.8;  %(tractor wheelbase)
L_1f = 7.21; %(trailer wheel base)
L_0b = 0.48;
        %updating the vehicle position to controller
                IC_x1= 0+Nn(1,1);                                                         % initial x-position of semi axle 
                IC_y1 = 0+Nn(1,2);
                IC_theta0 = Nn(1,4)+Nn(1,3);                                                   % initial yaw angle of tractor [deg]
                IC_theta1 = Nn(1,3);
                
                IC_x1f= L_1f*cos(IC_theta1)+IC_x1 ;                                                         % initial x-position of semi axle 
                IC_y1f =L_1f*sin(IC_theta1)+IC_y1 ;
                
                IC_x0f= (L_0f-L_0b)*cos(IC_theta0)+IC_x1f ;                                                         % initial x-position of semi axle 
                IC_y0f =(L_0f-L_0b)*sin(IC_theta0)+IC_y1f ;
                
                IC_x0 =   IC_x0f-L_0f*cos(IC_theta0);                                                           % initial x-position of tractor drive axle 
                IC_y0 =   IC_y0f-L_0f*sin(IC_theta0);

== matlab function clrrtsf/Chart/goalregion_reachability.goalregionreachability/wrapTo2Pi ==
  data: u input; y output
function y = fcn(u)
y=0;
coder.extrinsic('wrapTo2Pi')
y = wrapTo2Pi(u);
